simulink model "integrated_model"  (R2022a)
settings: Solver=FixedStepDiscrete  StartTime=0.0  StopTime=Inf  RelTol=1e-3  EnableMultiTasking=on
undefined symbols (not defined in the file or in its folder): Down, GPTRIP1SEL, GPTRIP2SEL, Hi, High, Impedance, parControl, parSimulacio, TZ1, TZ2, Up, Z
libraries: c2802xlib x10, simulink x9, c2837xDlib x6, c2000lib x1
(part 2 of 2)

== system integrated_model/Function-Call Subsystem/Switch Case Action Subsystem16 ==
  Action Port : ActionPort  ActionPortLabel=case [ 5 ]:
  Constant : Constant  Value=-1  OutDataTypeStr=single
  Constant2 : Constant  Value=45  OutDataTypeStr=single
  Divide : Product  Inputs=*/  RndMeth=Zero  SaturateOnIntegerOverflow=on
  Pi : Constant  Value=pi  OutDataTypeStr=single
  Product : Product
  Out1 : Outport  OutputWhenDisabled=reset  InitialOutput=0
  wires:
  Product/1 -> Out1/1
  Constant2/1 -> Divide/2
  Divide/1 -> Product/2
  Constant/1 -> Divide/1
  Pi/1 -> Product/1

== system integrated_model/Function-Call Subsystem/Switch Case Action Subsystem17 ==
  Inport : Inport
  Action Port : ActionPort  ActionPortLabel=default:
  Constant2 : Constant  Value=45  OutDataTypeStr=single
  Divide : Product  Inputs=*/  RndMeth=Zero  SaturateOnIntegerOverflow=on
  Pi : Constant  Value=pi  OutDataTypeStr=single
  Product : Product
  Out1 : Outport  OutputWhenDisabled=reset  InitialOutput=0
  wires:
  Product/1 -> Out1/1
  Constant2/1 -> Divide/2
  Divide/1 -> Product/2
  Inport/1 -> Divide/1
  Pi/1 -> Product/1

== system integrated_model/Function-Call Subsystem/Triggered Subsystem2 ==
  note: Limit angle between certain values
  Inport : Inport  OutDataTypeStr=single
  Trigger : TriggerPort  VariantControl=(inherit)
  Add : Sum
  Constant1 : Constant  Commented=on  Value=0  OutDataTypeStr=single
  Interval Test : simulink/Logic and Bit Operations/Interval Test  Commented=on  IntervalClosedRight=off  uplimit=2*pi  IntervalClosedLeft=off  lowlimit=0  OutDataTypeStr=boolean
  Memory : Memory  InheritSampleTime=on
  Switch : Switch  Commented=on  Criteria=u2 ~= 0  Threshold=90  OutDataTypeStr=single  SaturateOnIntegerOverflow=off  InputSameDT=off
  Outport : Outport  InitialOutput=0
  wires:
  Add/1 -> Outport/1, Memory/1
  Memory/1 -> Add/2
  Interval Test/1 -> Switch/2
  Constant1/1 -> Switch/3
  Inport/1 -> Add/1

== system integrated_model/Function-Call Subsystem/Triggered Subsystem3 ==
  In1 : Inport  LatchByDelayingOutsideSignal=on
  Inport : Inport  Port=2
  Trigger : TriggerPort  VariantControl=(inherit)
  Constant : Constant  Value=5000  OutDataTypeStr=single
  Data Store Write8 : DataStoreWrite  DataStoreName=MOT_VEL  IndexOptions=Index vector (dialog)  Indices=1  OutputSizes=1
  Divide : Product  Inputs=*/
  Divide1 : Product  Inputs=*/
  wires:
  In1/1 -> Divide/1
  Constant/1 -> Divide/2
  Divide/1 -> Divide1/2
  Inport/1 -> Divide1/1
  Divide1/1 -> Data Store Write8/1

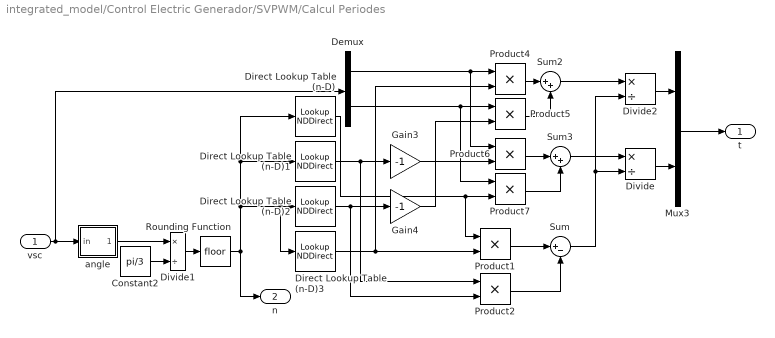
== system integrated_model/Control Electric Generador/SVPWM/Calcul Periodes ==
  vsc : Inport
  Constant2 : Constant  Value=pi/3  SampleTime=T
  Demux : Demux  Outputs=2
  Direct Lookup Table (n-D) : LookupNDDirect  NumberOfTableDimensions=1  Table=[2/3, 1/3, -1/3, -2/3, -1/3, 1/3]
  Direct Lookup Table (n-D)1 : LookupNDDirect  NumberOfTableDimensions=1  Table=[0, -sqrt(3)/3, -sqrt(3)/3, 0 ,sqrt(3)/3, sqrt(3)/3]
  Direct Lookup Table (n-D)2 : LookupNDDirect  NumberOfTableDimensions=1  Table=[1/3, -1/3, -2/3, -1/3, 1/3,2/3]
  Direct Lookup Table (n-D)3 : LookupNDDirect  NumberOfTableDimensions=1  Table=[-sqrt(3)/3, -sqrt(3)/3, 0 ,sqrt(3)/3, sqrt(3)/3,0]
  Divide : Product  Inputs=*/
  Divide1 : Product  Inputs=*/
  Divide2 : Product  Inputs=*/
  Gain3 : Gain  Gain=-1
  Gain4 : Gain  Gain=-1
  Mux3 : Mux  Inputs=2
  Product{1..2,4..7} (6 alike) : Product  RndMeth=Zero
  Rounding Function : Rounding
  Sum : Sum  Inputs=|+-
  Sum2 : Sum  Inputs=|++
  Sum3 : Sum  Inputs=|++
  angle : Subsystem
  t : Outport
  n : Outport  Port=2
  wires:
  angle/1(out) -> Divide1/1
  Constant2/1 -> Divide1/2
  Divide1/1 -> Rounding Function/1
  Rounding Function/1 -> n/1, Direct Lookup Table (n-D)1/1, Direct Lookup Table (n-D)/1, Direct Lookup Table (n-D)3/1, Direct Lookup Table (n-D)2/1
  vsc/1 -> angle/1(in), Demux/1
  Product1/1 -> Sum/1
  Product2/1 -> Sum/2
  Sum/1 -> Divide/2, Divide2/2
  Divide2/1 -> Mux3/1
  Divide/1 -> Mux3/2
  Mux3/1 -> t/1
  Product4/1 -> Sum2/1
  Product7/1 -> Sum3/2
  Sum3/1 -> Divide/1
  Sum2/1 -> Divide2/1
  Demux/1 -> Product4/1, Product6/1
  Demux/2 -> Product5/1, Product7/1
  Direct Lookup Table (n-D)3/1 -> Product4/2, Product1/2
  Direct Lookup Table (n-D)2/1 -> Product2/2, Gain4/1
  Gain4/1 -> Product5/2
  Direct Lookup Table (n-D)1/1 -> Gain3/1, Product2/1
  Gain3/1 -> Product6/2
  Direct Lookup Table (n-D)/1 -> Product7/2, Product1/1
  Product5/1 -> Sum2/2
  Product6/1 -> Sum3/1

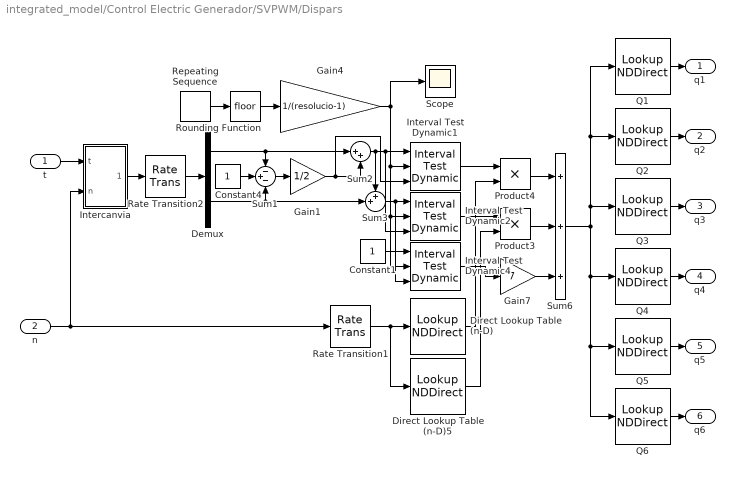
== system integrated_model/Control Electric Generador/SVPWM/Dispars ==
  t : Inport
  n : Inport  Port=2
  Constant1 : Constant  SampleTime=T/resolucio
  Constant4 : Constant  SampleTime=T/resolucio
  Demux : Demux  Outputs=2
  Direct Lookup Table (n-D) : LookupNDDirect  NumberOfTableDimensions=1  Table=[1,3,3,5,5,1]
  Direct Lookup Table (n-D)5 : LookupNDDirect  NumberOfTableDimensions=1  Table=[2,2,4,4,6,6]
  Gain1 : Gain  Gain=1/2  SampleTime=parControl.Electric.Generador.T/64
  Gain4 : Gain  Gain=1/(resolucio-1)  SampleTime=T/resolucio
  Gain7 : Gain  Gain=7
  Intercanvia : Subsystem
  Interval Test Dynamic1 : simulink/Logic and Bit Operations/Interval Test Dynamic  IntervalClosedRight=off  IntervalClosedLeft=on  OutDataTypeStr=uint8
      settings: SourceProductBaseCode=SL
  Interval Test Dynamic2 : simulink/Logic and Bit Operations/Interval Test Dynamic  IntervalClosedRight=off  IntervalClosedLeft=on  OutDataTypeStr=uint8
      settings: SourceProductBaseCode=SL
  Interval Test Dynamic4 : simulink/Logic and Bit Operations/Interval Test Dynamic  IntervalClosedRight=on  IntervalClosedLeft=on  OutDataTypeStr=uint8
      settings: SourceProductBaseCode=SL
  Product3 : Product  RndMeth=Zero
  Product4 : Product  RndMeth=Zero
  Q1 : LookupNDDirect  NumberOfTableDimensions=1  Table=[0,1,1,0,0,0,1,1]
  Q2 : LookupNDDirect  NumberOfTableDimensions=1  Table=[1,1,1,1,0,0,0,0]
  Q3 : LookupNDDirect  NumberOfTableDimensions=1  Table=[0,0,1,1,1,0,0,1]
  Q4 : LookupNDDirect  NumberOfTableDimensions=1  Table=[1,0,0,1,1,1,0,0]
  Q5 : LookupNDDirect  NumberOfTableDimensions=1  Table=[0,0,0,0,1,1,1,1]
  Q6 : LookupNDDirect  NumberOfTableDimensions=1  Table=[1,1,0,0,0,1,1,0]
  Rate Transition1 : RateTransition  OutPortSampleTime=T/resolucio
  Rate Transition2 : RateTransition  OutPortSampleTime=T/resolucio
  Repeating Sequence : simulink/Sources/Repeating Sequence  rep_seq_t=[0, T, 2*T]  rep_seq_y=[0,resolucio-1e-3,0]
  Rounding Function : Rounding
  Scope : Scope
  Sum1 : Sum  Inputs=-+-
  Sum2 : Sum  Inputs=|++
  Sum3 : Sum  Inputs=++|
  Sum6 : Sum  Inputs=+++
  q1 : Outport
  q2 : Outport  Port=2
  q3 : Outport  Port=3
  q4 : Outport  Port=4
  q5 : Outport  Port=5
  q6 : Outport  Port=6
  wires:
  Interval Test Dynamic1/1 -> Product4/1
  Interval Test Dynamic2/1 -> Product3/1
  Repeating Sequence/1 -> Rounding Function/1
  Gain4/1 -> Interval Test Dynamic1/2, Interval Test Dynamic2/2, Interval Test Dynamic4/2, Scope/1
  Constant4/1 -> Sum1/2
  Demux/1 -> Sum1/1, Sum2/1
  Demux/2 -> Sum1/3, Sum3/2
  Sum1/1 -> Gain1/1
  Gain1/1 -> Sum2/2, Interval Test Dynamic1/3
  Sum2/1 -> Sum3/1, Interval Test Dynamic1/1, Interval Test Dynamic2/3
  Sum3/1 -> Interval Test Dynamic2/1, Interval Test Dynamic4/3
  Constant1/1 -> Interval Test Dynamic4/1
  Product4/1 -> Sum6/1
  Product3/1 -> Sum6/2
  Gain7/1 -> Sum6/3
  Direct Lookup Table (n-D)/1 -> Product4/2
  Direct Lookup Table (n-D)5/1 -> Product3/2
  Sum6/1 -> Q1/1, Q2/1, Q3/1, Q4/1, Q5/1, Q6/1
  Q1/1 -> q1/1
  Q2/1 -> q2/1
  Q3/1 -> q3/1
  Q4/1 -> q4/1
  Q5/1 -> q5/1
  Q6/1 -> q6/1
  Rate Transition2/1 -> Demux/1
  Rounding Function/1 -> Gain4/1
  t/1 -> Intercanvia/1(t)
  Interval Test Dynamic4/1 -> Gain7/1
  n/1 -> Intercanvia/2(n), Rate Transition1/1
  Intercanvia/1(tswap) -> Rate Transition2/1
  Rate Transition1/1 -> Direct Lookup Table (n-D)/1, Direct Lookup Table (n-D)5/1

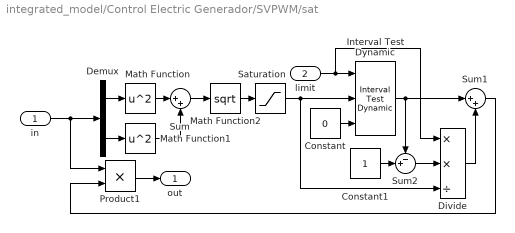
== system integrated_model/Control Electric Generador/SVPWM/sat ==
  in : Inport
  limit : Inport  Port=2
  Constant : Constant  Value=0  SampleTime=T
  Constant1 : Constant  SampleTime=T
  Demux : Demux  Outputs=2
  Divide : Product  Inputs=**/
  Interval Test Dynamic : simulink/Logic and Bit Operations/Interval Test Dynamic  IntervalClosedRight=on  IntervalClosedLeft=on  OutDataTypeStr=uint8
      settings: SourceProductBaseCode=SL
  Math Function : Math  Operator=square  SignedPower=on
  Math Function1 : Math  Operator=square  SignedPower=on
  Math Function2 : Math  Operator=sqrt  SignedPower=on
  Product1 : Product  RndMeth=Zero
  Saturation : Saturate  UpperLimit=inf  LowerLimit=1
  Sum : Sum  Inputs=|++
  Sum1 : Sum  Inputs=|++
  Sum2 : Sum  Inputs=-+|
  out : Outport
  wires:
  Math Function/1 -> Sum/1
  Math Function1/1 -> Sum/2
  Sum/1 -> Math Function2/1
  Math Function2/1 -> Saturation/1
  Demux/1 -> Math Function/1
  Demux/2 -> Math Function1/1
  in/1 -> Demux/1, Product1/1
  Product1/1 -> out/1
  Constant/1 -> Interval Test Dynamic/3
  Interval Test Dynamic/1 -> Sum1/1, Sum2/1
  Constant1/1 -> Sum2/2
  limit/1 -> Divide/1, Interval Test Dynamic/1
  Sum2/1 -> Divide/2
  Divide/1 -> Sum1/2
  Sum1/1 -> Product1/2
  Saturation/1 -> Divide/3, Interval Test Dynamic/2

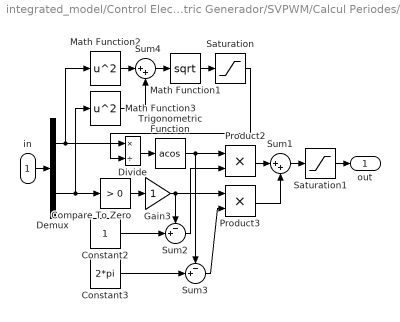
== system integrated_model/Control Electric Generador/SVPWM/Calcul Periodes/angle ==
  in : Inport
  Compare To Zero : simulink/Logic and Bit Operations/Compare To Zero  relop=>  OutDataTypeStr=uint8  ZeroCross=off
  Constant2 : Constant  SampleTime=T
  Constant3 : Constant  Value=2*pi  SampleTime=T
  Demux : Demux  Outputs=2
  Divide : Product  Inputs=*/
  Gain3 : Gain  SampleTime=T
  Math Function1 : Math  Operator=sqrt  SignedPower=on
  Math Function2 : Math  Operator=square  SignedPower=on
  Math Function3 : Math  Operator=square  SignedPower=on
  Product2 : Product  RndMeth=Zero
  Product3 : Product  RndMeth=Zero
  Saturation : Saturate  UpperLimit=inf  LowerLimit=1e-3
  Saturation1 : Saturate  UpperLimit=2*pi-1e-3  LowerLimit=0
  Sum1 : Sum  Inputs=|++
  Sum2 : Sum  Inputs=-+|
  Sum3 : Sum  Inputs=-+|
  Sum4 : Sum  Inputs=|++
  Trigonometric Function : Trigonometry  Operator=acos
  out : Outport
  wires:
  Demux/2 -> Compare To Zero/1, Math Function3/1
  Constant2/1 -> Sum2/2
  Compare To Zero/1 -> Gain3/1
  Trigonometric Function/1 -> Sum3/1, Product2/1
  Sum2/1 -> Product2/2
  Constant3/1 -> Sum3/2
  Sum3/1 -> Product3/2
  Product2/1 -> Sum1/1
  Product3/1 -> Sum1/2
  in/1 -> Demux/1
  Sum1/1 -> Saturation1/1
  Gain3/1 -> Sum2/1, Product3/1
  Divide/1 -> Trigonometric Function/1
  Demux/1 -> Math Function2/1, Divide/1
  Math Function2/1 -> Sum4/1
  Math Function3/1 -> Sum4/2
  Sum4/1 -> Math Function1/1
  Math Function1/1 -> Saturation/1
  Saturation/1 -> Divide/2
  Saturation1/1 -> out/1

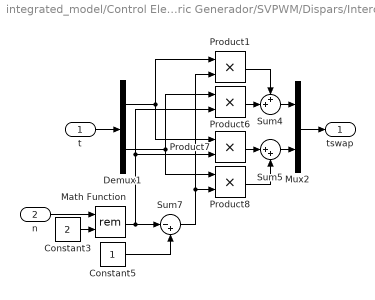
== system integrated_model/Control Electric Generador/SVPWM/Dispars/Intercanvia ==
  t : Inport
  n : Inport  Port=2
  Constant3 : Constant  Value=2  SampleTime=parControl.Electric.Generador.T/64
  Constant5 : Constant  SampleTime=parControl.Electric.Generador.T/64
  Demux1 : Demux  Outputs=2
  Math Function : Math  Operator=rem  SignedPower=on
  Mux2 : Mux  Inputs=2
  Product{1,6..8} (4 alike) : Product  RndMeth=Zero
  Sum4 : Sum  Inputs=++|
  Sum5 : Sum  Inputs=|++
  Sum7 : Sum  Inputs=|-+
  tswap : Outport
  wires:
  Sum4/1 -> Mux2/1
  Sum5/1 -> Mux2/2
  Product1/1 -> Sum4/1
  Product6/1 -> Sum4/2
  Product7/1 -> Sum5/1
  Product8/1 -> Sum5/2
  Demux1/1 -> Product1/1, Product7/1
  Demux1/2 -> Product6/1, Product8/1
  Constant3/1 -> Math Function/2
  Math Function/1 -> Sum7/1, Product6/2, Product7/2
  Constant5/1 -> Sum7/2
  n/1 -> Math Function/1
  t/1 -> Demux1/1
  Mux2/1 -> tswap/1
  Sum7/1 -> Product1/2, Product8/2
